simulink model "BLDC_180deg_compareModels"  (R2024a)
settings: Solver=ode15s  StartTime=0.0  StopTime=3.0  RelTol=1e-3
settings Model: Creator=matthewhasman  LastModifiedBy=matthewhasman

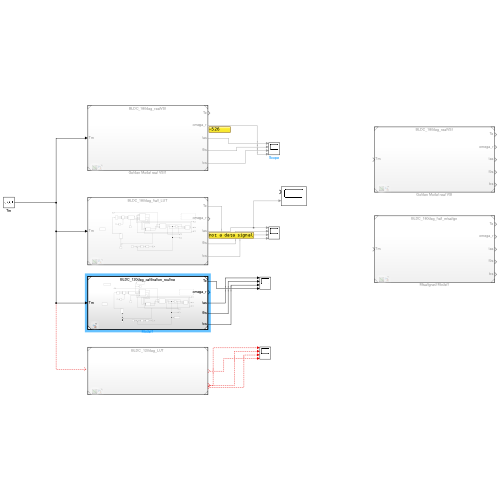
[thumbnail: Simulink's stored preview of the top-level diagram]
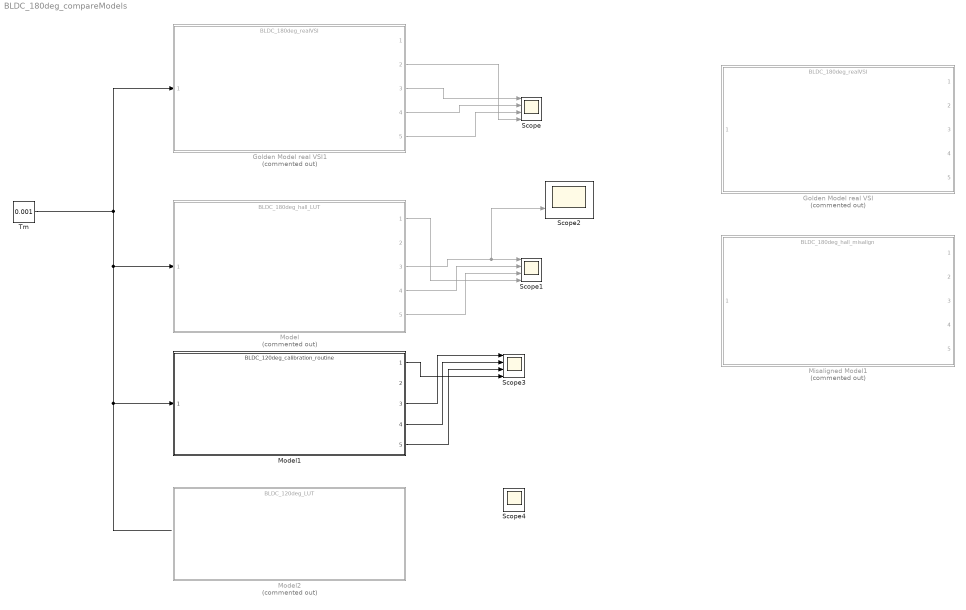
== system BLDC_180deg_compareModels ==
  Golden Model real VSI : ModelReference  Commented=on  ModelNameDialog=BLDC_180deg_realVSI.slx  SimulationMode=Normal  ModelReferenceVersion=1.74
  Golden Model real VSI1 : ModelReference  Commented=on  ModelNameDialog=BLDC_180deg_realVSI.slx  SimulationMode=Normal  ModelReferenceVersion=1.74
  Misaligned Model1 : ModelReference  Commented=on  ModelNameDialog=BLDC_180deg_hall_misalign.slx  SimulationMode=Normal  ModelReferenceVersion=1.127
  Model : ModelReference  Commented=on  ModelNameDialog=BLDC_180deg_hall_LUT.slx  SimulationMode=Normal  ModelReferenceVersion=1.172
  Model1 : ModelReference  ModelNameDialog=BLDC_120deg_calibration_routine.slx  SimulationMode=Normal  ModelReferenceVersion=1.180
  Model2 : ModelReference  Commented=on  ModelNameDialog=BLDC_120deg_LUT.slx  SimulationMode=Normal  ModelReferenceVersion=1.175
  Scope{,1,3..4} (4 alike) : Scope  NumInputPorts=4
  Scope2 : Scope  NumInputPorts=2
  Tm : Constant  Value=0.001
  wires:
  Tm/1 -> Model1/1, Model/1, Golden Model real VSI1/1
  Golden Model real VSI1/3 -> Scope/1
  Golden Model real VSI1/4 -> Scope/2
  Golden Model real VSI1/5 -> Scope/3
  Model/4 -> Scope1/2
  Model/5 -> Scope1/3
  Model/3 -> Scope2/2, Scope1/1
  Model/1 -> Scope1/4
  Model1/3 -> Scope3/1
  Model1/4 -> Scope3/2
  Model1/5 -> Scope3/3
  Model1/1 -> Scope3/4
  ? -> Scope4/4
  ? -> Scope4/1
  ? -> Scope4/2
  ? -> Scope4/3
  Golden Model real VSI1/2 -> Scope/4
